simulink model "cosine_trigger_6_pulse"  (R2025a)
settings: Solver=VariableStepAuto  StartTime=0.0  StopTime=3  RelTol=1e-3
libraries: simulink x6, spsCurrentMeasurementLib x1, spsSeriesRLCBranchLib x1, spsThreePhaseSourceLib x1, spsUniversalBridgeLib x1, spsVoltageMeasurementLib x1, sps_lib x1
settings Model: Creator=aditl  LastModifiedBy=aditl

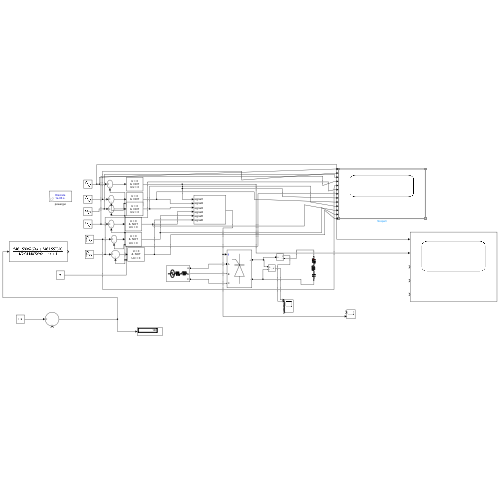
[thumbnail: Simulink's stored preview of the top-level diagram]
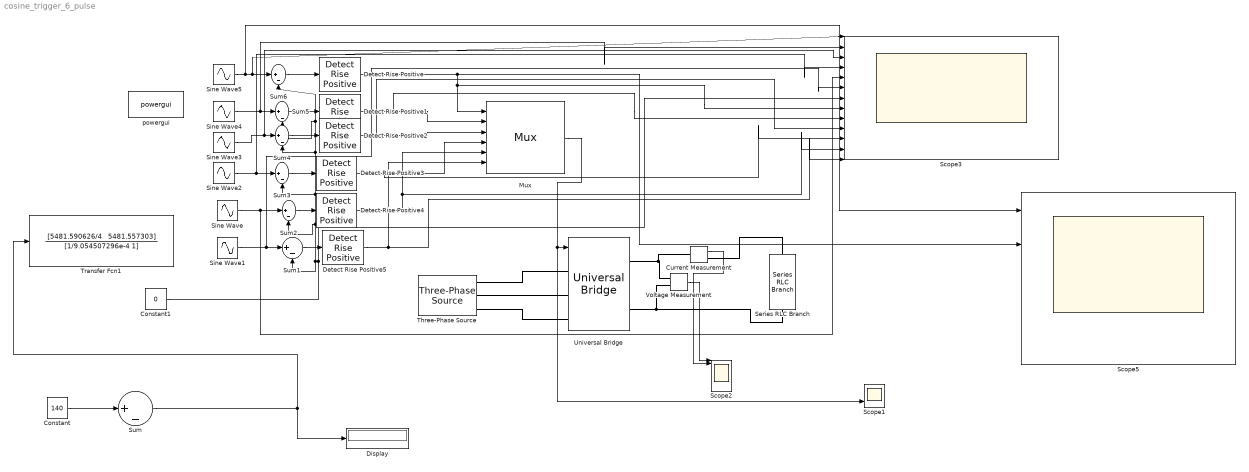
== system cosine_trigger_6_pulse ==
  Constant : Constant  Value=140  SampleTime=5e-5
  Constant1 : Constant  Value=0
  Current Measurement : spsCurrentMeasurementLib/Current Measurement  PhasorSimulation=off  OutputType=Complex  PSBequivalent=0
  Detect Rise Positive{,1..5} (6 alike) : simulink/Logic and Bit Operations/Detect Rise Positive  vinit=0  InputProcessing=Columns as channels (frame based)  OutDataTypeStr=boolean
  Display : Display
  Mux : Mux  Inputs=6
      settings: DisplayOption=signals
  Scope1 : Scope  NumInputPorts=2
      settings: ActiveDisplayYMinimum=-0.12499999999999997  ActiveDisplayYMaximum=1.125
  Scope2 : Scope  NumInputPorts=10
      settings: ActiveDisplayYMinimum=-3848.390229839998  ActiveDisplayYMaximum=4104.9520185879455  DataLoggingVariableName=ScopeData2
  Scope3 : Scope  NumInputPorts=13
      settings: ActiveDisplayYMinimum=-1249.9999999961581  ActiveDisplayYMaximum=1249.9999999673053  DataLoggingVariableName=ScopeData3
  Scope5 : Scope  NumInputPorts=5
      settings: ActiveDisplayYMinimum=-1249.9999999996196  ActiveDisplayYMaximum=1249.9999999976617  DataLoggingVariableName=ScopeData5
  Series RLC Branch : spsSeriesRLCBranchLib/Series RLC Branch  LConnTagsString=__new0  RConnTagsString=__new0  BranchType=RLC  Resistance=1  Inductance=100000  SetiL0=off  InitialCurrent=0  Capacitance=1e-6  Setx0=off  InitialVoltage=0  Measurements=None
  Sine Wave : Sin  Amplitude=1000  Frequency=5000  SampleTime=0
  Sine Wave1 : Sin  Amplitude=1000  Frequency=5000  Phase=pi/3  SampleTime=0
  Sine Wave2 : Sin  Amplitude=1000  Frequency=5000  Phase=-(pi/3)  SampleTime=0
  Sine Wave3 : Sin  Amplitude=1000  Frequency=5000  Phase=-(2*pi/3)  SampleTime=0
  Sine Wave4 : Sin  Amplitude=1000  Frequency=5000  Phase=-(3*pi/3)  SampleTime=0
  Sine Wave5 : Sin  Amplitude=1000  Frequency=5000  Phase=-(4*pi/3)  SampleTime=0
  Sum{,1..6} (7 alike) : Sum  Inputs=|+-
  Three-Phase Source : spsThreePhaseSourceLib/Three-Phase Source  InternalConnection=Y  VoltagePhases=off  Voltage=205.2079728  PhaseAngle=0  Voltage_phases=[25e3 25e3 25e3]/sqrt(3)  PhaseAngles_phases=[0 -120 +120]  Frequency=50  NonIdealSource=on  SpecifyImpedance=off  Resistance=0.8929  Inductance=16.58e-3  ShortCircuitLevel=100e6  BaseVoltage=25e3  XRratio=7  BusType=swing  Pref=10e3  Qref=0  Prefabc=[10e3, 10e3, 10e3]  Qrefabc=[0, 0, 0]  Qmin=-inf  Qmax=inf
  Transfer Fcn1 : TransferFcn  Numerator="[5481.590626/4   5481.557303]"  Denominator=[1/9.054507296e-4 1]  ParameterTunability=Unconstrained
  Universal Bridge : spsUniversalBridgeLib/Universal Bridge  Arms=3  SnubberResistance=1e5  SnubberCapacitance=inf  Device=Thyristors  Ron=1e-3  Lon=0  ForwardVoltages="[  0  0  ]"  ForwardVoltage=0  GTOparameters=[ 10e-6 , 20e-6 ]  IGBTparameters=[ 1e-6 , 2e-6 ]  Measurements=All voltages and currents  Measurements_2=None  converterType=Rectifier
  Voltage Measurement : spsVoltageMeasurementLib/Voltage Measurement  PhasorSimulation=off  OutputType=Complex  PSBequivalent=0
  powergui : sps_lib/powergui  Priority=1  SimulationMode=Discrete  SampleTime=1e-6  frequency=60  Iterations=50  frequencyindice=0  Pbase=100e6  ErrMax=1e-4  UnitsV=kV  UnitsW=MW  buscounter=0  FunctionMessages=off  echomessages=off  EnableUseOfTLC=off  CurrentSourceSwitches=off  DisableSnubberDevices=off  DisableRonSwitches=off  DisableVfSwitches=off  DisplayEquations=off  AutomaticDiscreteSolvers=off  SolverType=Tustin/Backward Euler (TBE)  Interpol=off  ExternalGateDelay=off  methode=off  Ts=100  x0status=blocks  SPID=on  SwTol=0  HookPort=off  NonlinearTolerance=1e-4  nMaxIteration=100  ContinueOnMaxIteration=off  RestoreLinks=warning  ResistiveCurrentMeasurement=off  Frange=[0:2:500]  Ylog=off  Xlog=on  ShowGrid=off  save=off  variable=ZData  structure=0  ZoomFFT=off  StartTime=0.0  cycles=1  DisplayStyle=1  fundamental=60  FreqAxis=off  MaxFrequency=1000  frequencyindicesteady=1  RmsSteady=1  display=off
  wires:
  Sum5/1 -> Detect Rise Positive1/1
  Detect Rise Positive/1 -> Scope5/2, Mux/1, Scope3/8
  Sum6/1 -> Detect Rise Positive/1
  Sum4/1 -> Detect Rise Positive2/1
  Sum1/1 -> Detect Rise Positive5/1
  Detect Rise Positive3/1 -> Scope3/11, Mux/4
  Detect Rise Positive5/1 -> Scope3/13, Mux/6
  Detect Rise Positive4/1 -> Scope3/12, Mux/5
  Sine Wave1/1 -> Scope3/6, Sum1/1
  Sine Wave4/1 -> Scope3/2, Sum5/1
  Mux/1 -> Universal Bridge/1, Scope1/2
  Sine Wave/1 -> Scope3/5, Sum2/1
  Constant1/1 -> Sum4/2, Sum5/2, Sum6/2, Sum3/2, Sum2/2, Sum1/2, Scope3/7
  Sum/1 -> Transfer Fcn1/1, Display/1
  Sine Wave3/1 -> Scope3/3, Sum4/1
  Sine Wave5/1 -> Scope5/1, Scope3/1, Sum6/1
  Sine Wave2/1 -> Scope3/4, Sum3/1
  Detect Rise Positive1/1 -> Scope3/9, Mux/2
  Detect Rise Positive2/1 -> Scope3/10, Mux/3
  Sum3/1 -> Detect Rise Positive3/1
  Sum2/1 -> Detect Rise Positive4/1
  Constant/1 -> Sum/1
  Voltage Measurement/1 -> Scope2/1
  Current Measurement/1 -> Scope2/2
  connections:
  Voltage Measurement/LConn1 -- Current Measurement/LConn1 -- Universal Bridge/RConn1
  Three-Phase Source/RConn1 -- Universal Bridge/LConn1
  Three-Phase Source/RConn3 -- Universal Bridge/LConn3
  Three-Phase Source/RConn2 -- Universal Bridge/LConn2
  Series RLC Branch/RConn1 -- Voltage Measurement/LConn2 -- Universal Bridge/RConn2
  Current Measurement/RConn1 -- Series RLC Branch/LConn1
